simulink model "controller_template"  (R2014a)
settings: Solver=FixedStepDiscrete  StartTime=0.0  StopTime=inf  FixedStep=sample_time  RelTol=1e-3
undefined symbols (not defined in the file or in its folder): control_start_time
libraries: simulink x1
settings Model: xpc_rtwmakecfg_data=_xpcethercatlib_  BufferReuse=off  Creator=wmartin  LastModifiedBy=wmartin
settings SolverCC: EnableConcurrentExecution=on
settings DataIOCC: MaxDataPoints=1000000000  SaveFormat=StructureWithTime
settings OptimizationCC: BlockReduction=off  OptimizeBlockIOStorage=off  BufferReuse=off  GlobalBufferReuse=off  ExpressionFolding=off  ExpressionDepthLimit=2147483647  LocalBlockOutputs=off  SimCompilerOptimization=On
settings DebuggingCC: UnderspecifiedInitializationDetection=Classic  StateNameClashWarn=warning
settings HardwareCC: ProdIntDivRoundTo=Zero  ProdEndianess=LittleEndian  ProdHWDeviceType=Generic->32-bit x86 compatible
settings ModelReferenceCC: UpdateModelReferenceTargets=IfOutOfDate  EnableParallelModelReferenceBuilds=on  ParallelModelReferenceMATLABWorkerInit=Copy Base Workspace
settings RTWCC: SystemTargetFile=slrt.tlc  TemplateMakefile=slrt_default_tmf  Description=Simulink Real-Time  RTWVerbose=off  ProcessScript=slrt_make_rtw_hook  RTWCompilerOptimization=On
settings CodeAppCC: MaxIdLength=127
settings SimulinkRealTimeCC: GeneratePreprocessorConditionals=Disable all  EnableShiftOperators=on  RL32LogBufSizeModifier=100000000

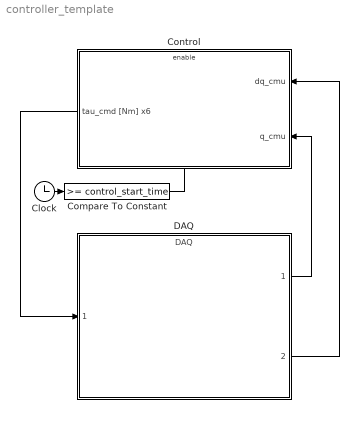
== system controller_template ==
  Clock : Clock
  Compare To Constant : simulink/Logic and Bit Operations/Compare To Constant  relop=>=  const=control_start_time  OutDataTypeStr=boolean
  Control : Subsystem
  DAQ : ModelReference  ModelNameDialog=DAQ  SimulationMode=Normal  ModelReferenceVersion=1.1653  CopyOfModelName=DAQ  DefaultDataLogging=on
  wires:
  DAQ/1 -> Control/2(q_cmu)
  DAQ/2 -> Control/1(dq_cmu)
  Clock/1 -> Compare To Constant/1
  Compare To Constant/1 -> Control/Enable
  Control/1(tau_cmd [Nm] x6) -> DAQ/1

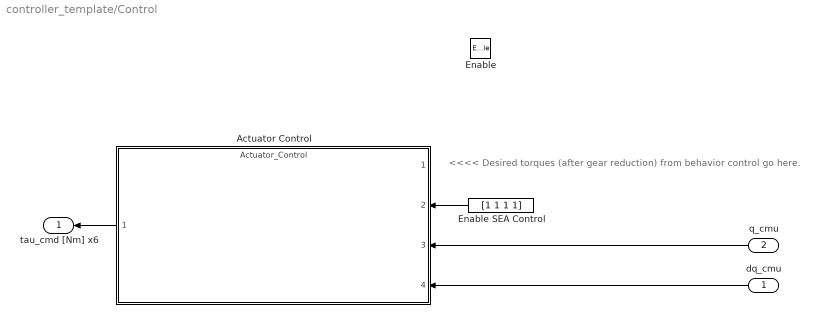
== system controller_template/Control ==
  note: <<<< Desired torques (after gear reduction) from behavior control go here.
  dq_cmu : Inport
  q_cmu : Inport  Port=2
  Enable : EnablePort  StatesWhenEnabling=reset
  Actuator Control : ModelReference  ModelNameDialog=Actuator_Control  SimulationMode=Normal  ModelReferenceVersion=1.16  CopyOfModelName=Actuator_Control  DefaultDataLogging=on
  Enable SEA Control : Constant  Value=[1 1 1 1]  OutDataTypeStr=boolean
  tau_cmd [Nm] x6 : Outport  InitialOutput=[0 0 0 0 0 0]
  wires:
  dq_cmu/1 -> Actuator Control/4
  Actuator Control/1 -> tau_cmd [Nm] x6/1
  q_cmu/1 -> Actuator Control/3
  Enable SEA Control/1 -> Actuator Control/2
